simulink model "fur_bring_down"  (R2015b)
settings: Solver=ode14x  StartTime=0.0  StopTime=inf  FixedStep=0.001  RelTol=1e-3
values from neighbouring files (symbols this model uses):
  A_aug = [A Bz; zeros(2,6)]    [Furuta_Pendulum_bring_down.m]    (also in Furuta_Pendulum_up_pos.m)
  B_aug = [B ;0;0]    [Furuta_Pendulum_bring_down.m]    (also in Furuta_Pendulum_up_pos.m)
  C_aug = [C zeros(2,2)]    [Furuta_Pendulum_bring_down.m]    (also in Furuta_Pendulum_up_pos.m)
  I_max = 0.5    [Furuta_Pendulum_bring_down.m]    (also in Furuta_Pendulum_up_pos.m = 0.8)
  Km = 7.86e-3    (= 0.00786)    [Furuta_Pendulum_bring_down.m]    (also in Furuta_Pendulum_up_pos.m)
  L_aug = real (L1+L2+L3)    [Furuta_Pendulum_bring_down.m]    (also in Furuta_Pendulum_up_pos.m)
  N = 70    [Furuta_Pendulum_bring_down.m]    (also in Furuta_Pendulum_up_pos.m)
  nu = 0.9    [Furuta_Pendulum_bring_down.m]    (also in Furuta_Pendulum_up_pos.m)
  Qz = - inv(Cr1*inv(Ar-Br*r')*Br)*Cr1*inv(Ar-Br*r')*Bzr    [Furuta_Pendulum_bring_down.m]    (also in Furuta_Pendulum_up_pos.m = inv(Cr1*inv(Ar-Br*r')*Br)*Cr1*inv(Ar-Br*r')*Bzr)
  R = 2.75    [Furuta_Pendulum_bring_down.m]    (also in Furuta_Pendulum_up_pos.m)
  Tr = [Su(end,:) ; Su(end,:)*A; Su(end,:)*A^2;Su(end,:)*A^3]    [Furuta_Pendulum_bring_down.m]    (also in Furuta_Pendulum_up_pos.m)
  V_max = 5    [Furuta_Pendulum_bring_down.m]    (also in Furuta_Pendulum_up_pos.m = 8)
undefined symbols (not defined in the file or in its folder): HIL
libraries: quarc_library x5
settings Model: SimulationMode=external  ExtModeTrigDuration=10000  Creator=sgillen  LastModifiedBy=sgillen
settings SolverCC: PositivePriorityOrder=on
settings RTWCC: SystemTargetFile=quarc_win64.tlc  TemplateMakefile=quarc_default_tmf  Description=QUARC Win64 Target
settings STFCustomTargetCC: GeneratePreprocessorConditionals=Use local settings  CPPClassGenCompliant=off
settings GRTTargetCC: ParMdlRefBuildCompliant=off  CompOptLevelCompliant=off  CombineOutputUpdateFcns=off  MatFileLogging=off  CPPClassGenCompliant=off  GRTInterface=on  UseToolchainInfoCompliant=off  ExtMode=on  ExtModeMexFile=quarc_comm

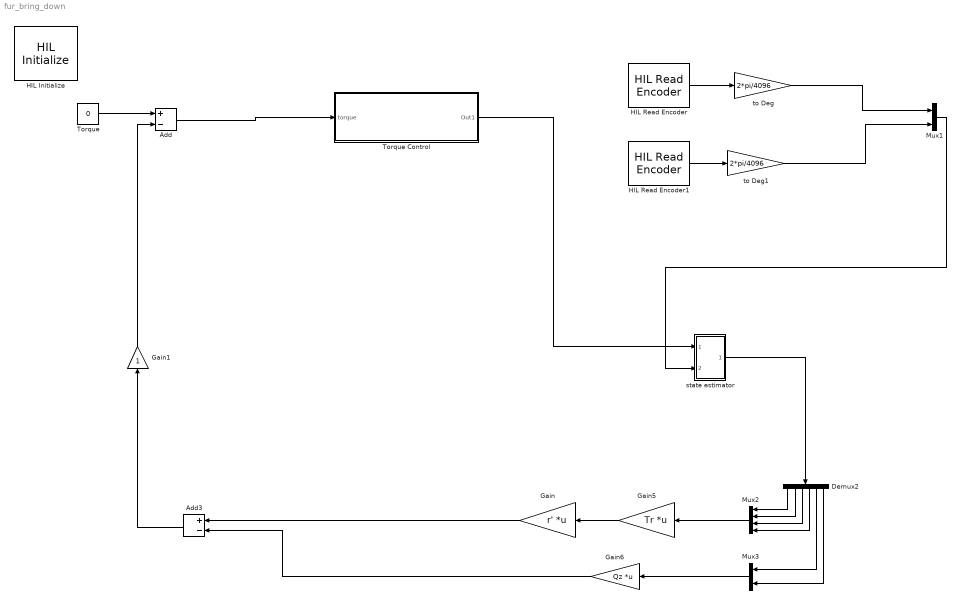
== system fur_bring_down ==
  Add : Sum  Inputs=+-
  Add3 : Sum  Inputs=+-
  Demux2 : Demux  Outputs=6
  Gain : Gain  Gain=r'  Multiplication=Matrix(K*u) (u vector)
  Gain1 : Gain
  Gain5 : Gain  Gain=Tr  Multiplication=Matrix(K*u) (u vector)
  Gain6 : Gain  Gain=Qz  Multiplication=Matrix(K*u) (u vector)
  HIL Initialize : quarc_library/Data Acquisition/Generic/Configuration/HIL Initialize  object_name=HIL-1  board_type=q4  board_number=0  board_options=""  exclusive=off  active=on  hardware_clocks=[0:1]  clock_modes=[0 0]  initial_clock_frequencies=[]  set_clock_params_at_start=on  set_clock_params_at_switch_in=off  set_clock_frequencies_at_start=off  set_clock_frequencies_at_switch_in=off  analog_input_channels=[0:3]  analog_input_configurations=[]  analog_input_maximums=10  analog_input_minimums=-10  set_analog_input_params_at_start=off  set_analog_input_params_at_switch_in=off  analog_output_channels=[0:3]  analog_output_maximums=[10]  analog_output_minimums=[-10]  initial_analog_outputs=[0]  final_analog_outputs=[0]  watchdog_analog_outputs=0  set_analog_output_params_at_start=on  set_analog_output_params_at_switch_in=off  set_analog_outputs_at_start=on  set_analog_outputs_at_switch_in=off  set_analog_outputs_at_terminate=on  set_analog_outputs_at_switch_out=off  set_analog_outputs_on_watchdog=off  digital_input_channels=[]  digital_output_channels=[]  digital_output_configuration=[]  initial_digital_outputs=[1]  final_digital_outputs=[1]  watchdog_digital_outputs=[2]  set_digital_output_params_at_start=off  set_digital_output_params_at_switch_in=off  set_digital_outputs_at_start=on  set_digital_outputs_at_switch_in=off  set_digital_outputs_at_terminate=on  set_digital_outputs_at_switch_out=off  set_digital_outputs_on_watchdog=off  encoder_channels=[0:3]  quadrature=[4]  encoder_filter_frequency=(1/60e-9)/1  initial_encoder_counts=[0]  set_encoder_params_at_start=on  set_encoder_params_at_switch_in=off  set_encoder_counts_at_start=on  set_encoder_counts_at_switch_in=off  pwm_channels=[]  pwm_modes=[0]  pwm_frequency=(1/60e-9)/1024  pwm_configuration=[]  pwm_alignment=[]  pwm_polarity=[]  pwm_leading_deadband=[]  pwm_trailing_deadband=[]  initial_pwm_outputs=[0]  final_pwm_outputs=[0]  watchdog_pwm_outputs=[]  set_pwm_params_at_start=on  set_pwm_params_at_switch_in=off  set_pwm_outputs_at_start=on  set_pwm_outputs_at_switch_in=off  set_pwm_outputs_at_terminate=on  set_pwm_outputs_at_switch_out=off  set_pwm_outputs_on_watchdog=off  other_output_channels=[]  initial_other_outputs=[]  final_other_outputs=[]  watchdog_other_outputs=[]  set_other_outputs_at_start=off  set_other_outputs_at_switch_in=off  set_other_outputs_at_terminate=off  set_other_outputs_at_switch_out=off  set_other_outputs_on_watchdog=off
  HIL Read Encoder : quarc_library/Data Acquisition/Generic/Immediate I//O/HIL Read Encoder  object_name=HIL-1  channels=0  sample_time=qc_get_step_size  active=on  vector_output=off  data_type_mode=Inherit via back propagation  data_type=double
  HIL Read Encoder1 : quarc_library/Data Acquisition/Generic/Immediate I//O/HIL Read Encoder  object_name=HIL-1  channels=1  sample_time=qc_get_step_size  active=on  vector_output=off  data_type_mode=Inherit via back propagation  data_type=double
  Mux1 : Mux  Inputs=2
  Mux2 : Mux
  Mux3 : Mux  Inputs=2
  Torque : Constant  Value=0
  Torque Control : Subsystem
  state estimator : Subsystem
  to Deg : Gain  Gain=2*pi/4096
  to Deg1 : Gain  Gain=2*pi/4096
  wires:
  HIL Read Encoder/1 -> to Deg/1
  HIL Read Encoder1/1 -> to Deg1/1
  to Deg1/1 -> Mux1/2
  to Deg/1 -> Mux1/1
  Demux2/1 -> Mux2/1
  Demux2/3 -> Mux2/3
  Demux2/2 -> Mux2/2
  Demux2/4 -> Mux2/4
  Demux2/5 -> Mux3/1
  Mux2/1 -> Gain5/1
  Gain5/1 -> Gain/1
  Gain/1 -> Add3/1
  Gain6/1 -> Add3/2
  Mux3/1 -> Gain6/1
  Demux2/6 -> Mux3/2
  Torque/1 -> Add/1
  Add/1 -> Torque Control/1(torque)
  Add3/1 -> Gain1/1
  Gain1/1 -> Add/2
  Torque Control/1(Out1) -> state estimator/1(In1)
  Mux1/1 -> state estimator/2(In2)
  state estimator/1(Out1) -> Demux2/1

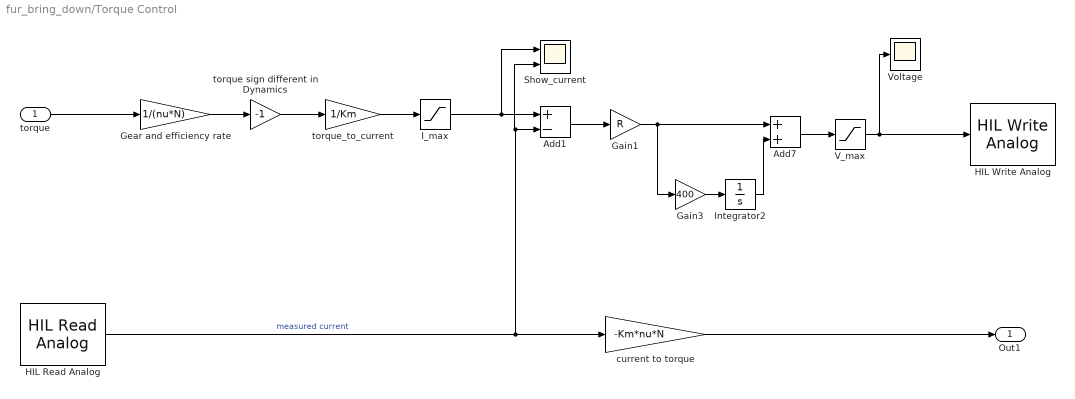
== system fur_bring_down/Torque Control ==
  torque : Inport
  Add1 : Sum  Inputs=+-
  Add7 : Sum
  Gain1 : Gain  Gain=R
  Gain3 : Gain  Gain=400
  Gear and efficiency rate : Gain  Gain=1/(nu*N)
  HIL Read Analog : quarc_library/Data Acquisition/Generic/Immediate I//O/HIL Read Analog  object_name=HIL-1  channels=1  sample_time=qc_get_step_size  active=on  vector_output=off
  HIL Write Analog : quarc_library/Data Acquisition/Generic/Immediate I//O/HIL Write Analog  object_name=HIL-1  channels=0  sample_time=-1  active=off  vector_input=off
  I_max : Saturate  UpperLimit=I_max  LowerLimit=-I_max
  Integrator2 : Integrator
  Show_current : Scope  NumInputPorts=2
  V_max : Saturate  UpperLimit=V_max  LowerLimit=-V_max
  Voltage : Scope
  current to torque : Gain  Gain=-Km*nu*N
  torque sign different in Dynamics : Gain  Gain=-1
  torque_to_current : Gain  Gain=1/Km
  Out1 : Outport
  wires:
  Gear and efficiency rate/1 -> torque sign different in Dynamics/1
  HIL Read Analog/1 -> Add1/2, Show_current/2, current to torque/1  "measured current"
  Add1/1 -> Gain1/1
  torque sign different in Dynamics/1 -> torque_to_current/1
  Add7/1 -> V_max/1
  I_max/1 -> Show_current/1, Add1/1
  Gain3/1 -> Integrator2/1
  Gain1/1 -> Add7/1, Gain3/1
  V_max/1 -> Voltage/1, HIL Write Analog/1
  Integrator2/1 -> Add7/2
  torque_to_current/1 -> I_max/1
  current to torque/1 -> Out1/1
  torque/1 -> Gear and efficiency rate/1

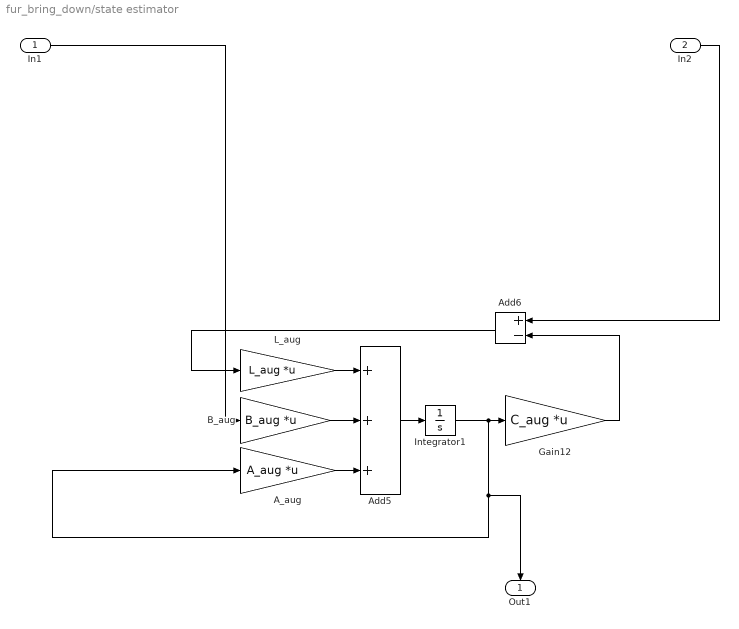
== system fur_bring_down/state estimator ==
  In1 : Inport
  In2 : Inport  Port=2
  A_aug : Gain  Gain=A_aug  Multiplication=Matrix(K*u) (u vector)
  Add5 : Sum  Inputs=+++
  Add6 : Sum  Inputs=+-
  B_aug : Gain  Gain=B_aug  Multiplication=Matrix(K*u) (u vector)
  Gain12 : Gain  Gain=C_aug  Multiplication=Matrix(K*u) (u vector)
  Integrator1 : Integrator
  "L_aug " : Gain  Gain=L_aug  Multiplication=Matrix(K*u) (u vector)
  Out1 : Outport
  wires:
  Integrator1/1 -> Gain12/1, Out1/1, A_aug/1
  Add5/1 -> Integrator1/1
  In2/1 -> Add6/1
  Gain12/1 -> Add6/2
  Add6/1 -> "L_aug "/1
  A_aug/1 -> Add5/3
  B_aug/1 -> Add5/2
  "L_aug "/1 -> Add5/1
  In1/1 -> B_aug/1
